simulink model "ieee80211n"  (Simulink 6.0)
settings: Solver=VariableStepDiscrete  StartTime=0.0  StopTime=inf  RelTol=1e-3
PreLoadFcn:
  | load IEEE80211n_init;
values from neighbouring files (symbols this model uses):
  params =     [IEEE80211n_init.mat]    (also in IEEE80211n_settings.m = p)
undefined symbols (not defined in the file or in its folder): magnitude
libraries: commblkintrlv2 x196, dspsigops x143, simulink x136, commdigbbndam2 x98, dspmtrx3 x96, dspsigattribs x69, dspstat3 x38, commutil2 x32, commsequence2 x26, commcnvcod2 x10, dspindex x9, dspmlti3 x8
(part 10 of 12)

== system ieee80211n/ModulatorBank/ModulatorSS1/Modulator 6 ==
  txdata : Inport  Port=1  LatchInput=off
  Enable : EnablePort
  Gain1 : Gain  SaturateOnIntegerOverflow=on
  General Block Interleaver : commblkintrlv2/General Block Interleaver  elements=interleaverElements
  Matrix Interleaver : commblkintrlv2/Matrix Interleaver  Nrows=interleaverRows  Ncols=interleaverCols
  Rectangular QAM Modulator Baseband : commdigbbndam2/Rectangular QAM Modulator Baseband  M=modOrder  InType=Bit  Enc=Gray  PowType=Average Power  MinDist=2  AvgPow=1  PeakPow=1  Ph=0  numSamp=1
  Zero Pad : dspsigops/Zero Pad  padSigAt=End  zpadAlong=Columns  padNumOutRowsSpecMethod=User-specified  numOutRows=Nb  padNumOutColsSpecMethod=User-specified  numOutCols=1  trunc_flag=None
      settings: AttributesFormatString=\n
  txsig : Outport
  wires:
  Rectangular QAM Modulator Baseband/1 -> Gain1/1
  Gain1/1 -> txsig/1
  txdata/1 -> Zero Pad/1
  Zero Pad/1 -> Matrix Interleaver/1
  Matrix Interleaver/1 -> General Block Interleaver/1
  General Block Interleaver/1 -> Rectangular QAM Modulator Baseband/1

== system ieee80211n/ModulatorBank/ModulatorSS1/Modulator 7 ==
  txdata : Inport  Port=1  LatchInput=off
  Enable : EnablePort
  Gain1 : Gain  SaturateOnIntegerOverflow=on
  General Block Interleaver : commblkintrlv2/General Block Interleaver  elements=interleaverElements
  Matrix Interleaver : commblkintrlv2/Matrix Interleaver  Nrows=interleaverRows  Ncols=interleaverCols
  Rectangular QAM Modulator Baseband : commdigbbndam2/Rectangular QAM Modulator Baseband  M=modOrder  InType=Bit  Enc=Gray  PowType=Average Power  MinDist=2  AvgPow=1  PeakPow=1  Ph=0  numSamp=1
  Zero Pad : dspsigops/Zero Pad  padSigAt=End  zpadAlong=Columns  padNumOutRowsSpecMethod=User-specified  numOutRows=Nb  padNumOutColsSpecMethod=User-specified  numOutCols=1  trunc_flag=None
      settings: AttributesFormatString=\n
  txsig : Outport
  wires:
  Rectangular QAM Modulator Baseband/1 -> Gain1/1
  Gain1/1 -> txsig/1
  txdata/1 -> Zero Pad/1
  Zero Pad/1 -> Matrix Interleaver/1
  Matrix Interleaver/1 -> General Block Interleaver/1
  General Block Interleaver/1 -> Rectangular QAM Modulator Baseband/1

== system ieee80211n/ModulatorBank/ModulatorSS1/Modulator 8 ==
  txdata : Inport  Port=1  LatchInput=off
  Enable : EnablePort
  Gain1 : Gain  SaturateOnIntegerOverflow=on
  General Block Interleaver : commblkintrlv2/General Block Interleaver  elements=interleaverElements
  Matrix Interleaver : commblkintrlv2/Matrix Interleaver  Nrows=interleaverRows  Ncols=interleaverCols
  Rectangular QAM Modulator Baseband : commdigbbndam2/Rectangular QAM Modulator Baseband  M=modOrder  InType=Bit  Enc=Gray  PowType=Average Power  MinDist=2  AvgPow=1  PeakPow=1  Ph=0  numSamp=1
  Zero Pad : dspsigops/Zero Pad  padSigAt=End  zpadAlong=Columns  padNumOutRowsSpecMethod=User-specified  numOutRows=Nb  padNumOutColsSpecMethod=User-specified  numOutCols=1  trunc_flag=None
      settings: AttributesFormatString=\n
  txsig : Outport
  wires:
  Rectangular QAM Modulator Baseband/1 -> Gain1/1
  Gain1/1 -> txsig/1
  txdata/1 -> Zero Pad/1
  Zero Pad/1 -> Matrix Interleaver/1
  Matrix Interleaver/1 -> General Block Interleaver/1
  General Block Interleaver/1 -> Rectangular QAM Modulator Baseband/1

== system ieee80211n/ModulatorBank/ModulatorSS2/Modulator 1 ==
  txdata : Inport  Port=1  LatchInput=off
  Enable : EnablePort
  Gain1 : Gain  SaturateOnIntegerOverflow=on
  General Block Interleaver : commblkintrlv2/General Block Interleaver  elements=interleaverElements
  General Block Interleaver1 : S-Function  AncestorBlock=commblkintrlv2/General Block Interleaver  FunctionName=scominterl  Parameters=elements,method  mask(General Block Interleaver){elements=freqRotInterleaverElements}
      mask help: Reorder the elements of the input vector. y = u(Elements). The length of Elements must match the input signal width.
      mask init:
      | method = 1;
      | commblkinterl(elements);
      mask Help: helpview(commbhelp)
      mask Display: disp('Frequency\nRotation\nInterleaver')
  Matrix Interleaver : commblkintrlv2/Matrix Interleaver  Nrows=interleaverRows  Ncols=interleaverCols
  Rectangular QAM Modulator Baseband : commdigbbndam2/Rectangular QAM Modulator Baseband  M=modOrder  InType=Bit  Enc=Gray  PowType=Average Power  MinDist=2  AvgPow=1  PeakPow=1  Ph=0  numSamp=1
  Zero Pad : dspsigops/Zero Pad  padSigAt=End  zpadAlong=Columns  padNumOutRowsSpecMethod=User-specified  numOutRows=Nb  padNumOutColsSpecMethod=User-specified  numOutCols=1  trunc_flag=None
      settings: AttributesFormatString=\n
  txsig : Outport
  wires:
  Rectangular QAM Modulator Baseband/1 -> Gain1/1
  Gain1/1 -> txsig/1
  txdata/1 -> Zero Pad/1
  Zero Pad/1 -> Matrix Interleaver/1
  Matrix Interleaver/1 -> General Block Interleaver/1
  General Block Interleaver/1 -> General Block Interleaver1/1
  General Block Interleaver1/1 -> Rectangular QAM Modulator Baseband/1

== system ieee80211n/ModulatorBank/ModulatorSS2/Modulator 2 ==
  txdata : Inport  Port=1  LatchInput=off
  Enable : EnablePort
  Gain1 : Gain  SaturateOnIntegerOverflow=on
  General Block Interleaver : commblkintrlv2/General Block Interleaver  elements=interleaverElements
  General Block Interleaver1 : S-Function  AncestorBlock=commblkintrlv2/General Block Interleaver  FunctionName=scominterl  Parameters=elements,method  mask(General Block Interleaver){elements=freqRotInterleaverElements}
      mask help: Reorder the elements of the input vector. y = u(Elements). The length of Elements must match the input signal width.
      mask init:
      | method = 1;
      | commblkinterl(elements);
      mask Help: helpview(commbhelp)
      mask Display: disp('Frequency\nRotation\nInterleaver')
  Matrix Interleaver : commblkintrlv2/Matrix Interleaver  Nrows=interleaverRows  Ncols=interleaverCols
  Rectangular QAM Modulator Baseband : commdigbbndam2/Rectangular QAM Modulator Baseband  M=modOrder  InType=Bit  Enc=Gray  PowType=Average Power  MinDist=2  AvgPow=1  PeakPow=1  Ph=0  numSamp=1
  Zero Pad : dspsigops/Zero Pad  padSigAt=End  zpadAlong=Columns  padNumOutRowsSpecMethod=User-specified  numOutRows=Nb  padNumOutColsSpecMethod=User-specified  numOutCols=1  trunc_flag=None
      settings: AttributesFormatString=\n
  txsig : Outport
  wires:
  Rectangular QAM Modulator Baseband/1 -> Gain1/1
  Gain1/1 -> txsig/1
  txdata/1 -> Zero Pad/1
  Zero Pad/1 -> Matrix Interleaver/1
  Matrix Interleaver/1 -> General Block Interleaver/1
  General Block Interleaver/1 -> General Block Interleaver1/1
  General Block Interleaver1/1 -> Rectangular QAM Modulator Baseband/1

== system ieee80211n/ModulatorBank/ModulatorSS2/Modulator 3 ==
  txdata : Inport  Port=1  LatchInput=off
  Enable : EnablePort
  Gain1 : Gain  SaturateOnIntegerOverflow=on
  General Block Interleaver : commblkintrlv2/General Block Interleaver  elements=interleaverElements
  General Block Interleaver1 : S-Function  AncestorBlock=commblkintrlv2/General Block Interleaver  FunctionName=scominterl  Parameters=elements,method  mask(General Block Interleaver){elements=freqRotInterleaverElements}
      mask help: Reorder the elements of the input vector. y = u(Elements). The length of Elements must match the input signal width.
      mask init:
      | method = 1;
      | commblkinterl(elements);
      mask Help: helpview(commbhelp)
      mask Display: disp('Frequency\nRotation\nInterleaver')
  Matrix Interleaver : commblkintrlv2/Matrix Interleaver  Nrows=interleaverRows  Ncols=interleaverCols
  Rectangular QAM Modulator Baseband : commdigbbndam2/Rectangular QAM Modulator Baseband  M=modOrder  InType=Bit  Enc=Gray  PowType=Average Power  MinDist=2  AvgPow=1  PeakPow=1  Ph=0  numSamp=1
  Zero Pad : dspsigops/Zero Pad  padSigAt=End  zpadAlong=Columns  padNumOutRowsSpecMethod=User-specified  numOutRows=Nb  padNumOutColsSpecMethod=User-specified  numOutCols=1  trunc_flag=None
      settings: AttributesFormatString=\n
  txsig : Outport
  wires:
  Rectangular QAM Modulator Baseband/1 -> Gain1/1
  Gain1/1 -> txsig/1
  txdata/1 -> Zero Pad/1
  Zero Pad/1 -> Matrix Interleaver/1
  Matrix Interleaver/1 -> General Block Interleaver/1
  General Block Interleaver/1 -> General Block Interleaver1/1
  General Block Interleaver1/1 -> Rectangular QAM Modulator Baseband/1

== system ieee80211n/ModulatorBank/ModulatorSS2/Modulator 4 ==
  txdata : Inport  Port=1  LatchInput=off
  Enable : EnablePort
  Gain1 : Gain  SaturateOnIntegerOverflow=on
  General Block Interleaver : commblkintrlv2/General Block Interleaver  elements=interleaverElements
  General Block Interleaver1 : S-Function  AncestorBlock=commblkintrlv2/General Block Interleaver  FunctionName=scominterl  Parameters=elements,method  mask(General Block Interleaver){elements=freqRotInterleaverElements}
      mask help: Reorder the elements of the input vector. y = u(Elements). The length of Elements must match the input signal width.
      mask init:
      | method = 1;
      | commblkinterl(elements);
      mask Help: helpview(commbhelp)
      mask Display: disp('Frequency\nRotation\nInterleaver')
  Matrix Interleaver : commblkintrlv2/Matrix Interleaver  Nrows=interleaverRows  Ncols=interleaverCols
  Rectangular QAM Modulator Baseband : commdigbbndam2/Rectangular QAM Modulator Baseband  M=modOrder  InType=Bit  Enc=Gray  PowType=Average Power  MinDist=2  AvgPow=1  PeakPow=1  Ph=0  numSamp=1
  Zero Pad : dspsigops/Zero Pad  padSigAt=End  zpadAlong=Columns  padNumOutRowsSpecMethod=User-specified  numOutRows=Nb  padNumOutColsSpecMethod=User-specified  numOutCols=1  trunc_flag=None
      settings: AttributesFormatString=\n
  txsig : Outport
  wires:
  Rectangular QAM Modulator Baseband/1 -> Gain1/1
  Gain1/1 -> txsig/1
  txdata/1 -> Zero Pad/1
  Zero Pad/1 -> Matrix Interleaver/1
  Matrix Interleaver/1 -> General Block Interleaver/1
  General Block Interleaver/1 -> General Block Interleaver1/1
  General Block Interleaver1/1 -> Rectangular QAM Modulator Baseband/1

== system ieee80211n/ModulatorBank/ModulatorSS2/Modulator 5 ==
  txdata : Inport  Port=1  LatchInput=off
  Enable : EnablePort
  Gain1 : Gain  SaturateOnIntegerOverflow=on
  General Block Interleaver : commblkintrlv2/General Block Interleaver  elements=interleaverElements
  General Block Interleaver1 : S-Function  AncestorBlock=commblkintrlv2/General Block Interleaver  FunctionName=scominterl  Parameters=elements,method  mask(General Block Interleaver){elements=freqRotInterleaverElements}
      mask help: Reorder the elements of the input vector. y = u(Elements). The length of Elements must match the input signal width.
      mask init:
      | method = 1;
      | commblkinterl(elements);
      mask Help: helpview(commbhelp)
      mask Display: disp('Frequency\nRotation\nInterleaver')
  Matrix Interleaver : commblkintrlv2/Matrix Interleaver  Nrows=interleaverRows  Ncols=interleaverCols
  Rectangular QAM Modulator Baseband : commdigbbndam2/Rectangular QAM Modulator Baseband  M=modOrder  InType=Bit  Enc=Gray  PowType=Average Power  MinDist=2  AvgPow=1  PeakPow=1  Ph=0  numSamp=1
  Zero Pad : dspsigops/Zero Pad  padSigAt=End  zpadAlong=Columns  padNumOutRowsSpecMethod=User-specified  numOutRows=Nb  padNumOutColsSpecMethod=User-specified  numOutCols=1  trunc_flag=None
      settings: AttributesFormatString=\n
  txsig : Outport
  wires:
  Rectangular QAM Modulator Baseband/1 -> Gain1/1
  Gain1/1 -> txsig/1
  txdata/1 -> Zero Pad/1
  Zero Pad/1 -> Matrix Interleaver/1
  Matrix Interleaver/1 -> General Block Interleaver/1
  General Block Interleaver/1 -> General Block Interleaver1/1
  General Block Interleaver1/1 -> Rectangular QAM Modulator Baseband/1

== system ieee80211n/ModulatorBank/ModulatorSS2/Modulator 6 ==
  txdata : Inport  Port=1  LatchInput=off
  Enable : EnablePort
  Gain1 : Gain  SaturateOnIntegerOverflow=on
  General Block Interleaver : commblkintrlv2/General Block Interleaver  elements=interleaverElements
  General Block Interleaver1 : S-Function  AncestorBlock=commblkintrlv2/General Block Interleaver  FunctionName=scominterl  Parameters=elements,method  mask(General Block Interleaver){elements=freqRotInterleaverElements}
      mask help: Reorder the elements of the input vector. y = u(Elements). The length of Elements must match the input signal width.
      mask init:
      | method = 1;
      | commblkinterl(elements);
      mask Help: helpview(commbhelp)
      mask Display: disp('Frequency\nRotation\nInterleaver')
  Matrix Interleaver : commblkintrlv2/Matrix Interleaver  Nrows=interleaverRows  Ncols=interleaverCols
  Rectangular QAM Modulator Baseband : commdigbbndam2/Rectangular QAM Modulator Baseband  M=modOrder  InType=Bit  Enc=Gray  PowType=Average Power  MinDist=2  AvgPow=1  PeakPow=1  Ph=0  numSamp=1
  Zero Pad : dspsigops/Zero Pad  padSigAt=End  zpadAlong=Columns  padNumOutRowsSpecMethod=User-specified  numOutRows=Nb  padNumOutColsSpecMethod=User-specified  numOutCols=1  trunc_flag=None
      settings: AttributesFormatString=\n
  txsig : Outport
  wires:
  Rectangular QAM Modulator Baseband/1 -> Gain1/1
  Gain1/1 -> txsig/1
  txdata/1 -> Zero Pad/1
  Zero Pad/1 -> Matrix Interleaver/1
  Matrix Interleaver/1 -> General Block Interleaver/1
  General Block Interleaver/1 -> General Block Interleaver1/1
  General Block Interleaver1/1 -> Rectangular QAM Modulator Baseband/1

== system ieee80211n/ModulatorBank/ModulatorSS2/Modulator 7 ==
  txdata : Inport  Port=1  LatchInput=off
  Enable : EnablePort
  Gain1 : Gain  SaturateOnIntegerOverflow=on
  General Block Interleaver : commblkintrlv2/General Block Interleaver  elements=interleaverElements
  General Block Interleaver1 : S-Function  AncestorBlock=commblkintrlv2/General Block Interleaver  FunctionName=scominterl  Parameters=elements,method  mask(General Block Interleaver){elements=freqRotInterleaverElements}
      mask help: Reorder the elements of the input vector. y = u(Elements). The length of Elements must match the input signal width.
      mask init:
      | method = 1;
      | commblkinterl(elements);
      mask Help: helpview(commbhelp)
      mask Display: disp('Frequency\nRotation\nInterleaver')
  Matrix Interleaver : commblkintrlv2/Matrix Interleaver  Nrows=interleaverRows  Ncols=interleaverCols
  Rectangular QAM Modulator Baseband : commdigbbndam2/Rectangular QAM Modulator Baseband  M=modOrder  InType=Bit  Enc=Gray  PowType=Average Power  MinDist=2  AvgPow=1  PeakPow=1  Ph=0  numSamp=1
  Zero Pad : dspsigops/Zero Pad  padSigAt=End  zpadAlong=Columns  padNumOutRowsSpecMethod=User-specified  numOutRows=Nb  padNumOutColsSpecMethod=User-specified  numOutCols=1  trunc_flag=None
      settings: AttributesFormatString=\n
  txsig : Outport
  wires:
  Rectangular QAM Modulator Baseband/1 -> Gain1/1
  Gain1/1 -> txsig/1
  txdata/1 -> Zero Pad/1
  Zero Pad/1 -> Matrix Interleaver/1
  Matrix Interleaver/1 -> General Block Interleaver/1
  General Block Interleaver/1 -> General Block Interleaver1/1
  General Block Interleaver1/1 -> Rectangular QAM Modulator Baseband/1

== system ieee80211n/ModulatorBank/ModulatorSS2/Modulator 8 ==
  txdata : Inport  Port=1  LatchInput=off
  Enable : EnablePort
  Gain1 : Gain  SaturateOnIntegerOverflow=on
  General Block Interleaver : commblkintrlv2/General Block Interleaver  elements=interleaverElements
  General Block Interleaver1 : S-Function  AncestorBlock=commblkintrlv2/General Block Interleaver  FunctionName=scominterl  Parameters=elements,method  mask(General Block Interleaver){elements=freqRotInterleaverElements}
      mask help: Reorder the elements of the input vector. y = u(Elements). The length of Elements must match the input signal width.
      mask init:
      | method = 1;
      | commblkinterl(elements);
      mask Help: helpview(commbhelp)
      mask Display: disp('Frequency\nRotation\nInterleaver')
  Matrix Interleaver : commblkintrlv2/Matrix Interleaver  Nrows=interleaverRows  Ncols=interleaverCols
  Rectangular QAM Modulator Baseband : commdigbbndam2/Rectangular QAM Modulator Baseband  M=modOrder  InType=Bit  Enc=Gray  PowType=Average Power  MinDist=2  AvgPow=1  PeakPow=1  Ph=0  numSamp=1
  Zero Pad : dspsigops/Zero Pad  padSigAt=End  zpadAlong=Columns  padNumOutRowsSpecMethod=User-specified  numOutRows=Nb  padNumOutColsSpecMethod=User-specified  numOutCols=1  trunc_flag=None
      settings: AttributesFormatString=\n
  txsig : Outport
  wires:
  Rectangular QAM Modulator Baseband/1 -> Gain1/1
  Gain1/1 -> txsig/1
  txdata/1 -> Zero Pad/1
  Zero Pad/1 -> Matrix Interleaver/1
  Matrix Interleaver/1 -> General Block Interleaver/1
  General Block Interleaver/1 -> General Block Interleaver1/1
  General Block Interleaver1/1 -> Rectangular QAM Modulator Baseband/1

== system ieee80211n/ModulatorBank/ModulatorSS3/Modulator 1 ==
  txdata : Inport  Port=1  LatchInput=off
  Enable : EnablePort
  Gain1 : Gain  SaturateOnIntegerOverflow=on
  General Block Interleaver : commblkintrlv2/General Block Interleaver  elements=interleaverElements
  General Block Interleaver1 : S-Function  AncestorBlock=commblkintrlv2/General Block Interleaver  FunctionName=scominterl  Parameters=elements,method  mask(General Block Interleaver){elements=freqRotInterleaverElements}
      mask help: Reorder the elements of the input vector. y = u(Elements). The length of Elements must match the input signal width.
      mask init:
      | method = 1;
      | commblkinterl(elements);
      mask Help: helpview(commbhelp)
      mask Display: disp('Frequency\nRotation\nInterleaver')
  Matrix Interleaver : commblkintrlv2/Matrix Interleaver  Nrows=interleaverRows  Ncols=interleaverCols
  Rectangular QAM Modulator Baseband : commdigbbndam2/Rectangular QAM Modulator Baseband  M=modOrder  InType=Bit  Enc=Gray  PowType=Average Power  MinDist=2  AvgPow=1  PeakPow=1  Ph=0  numSamp=1
  Zero Pad : dspsigops/Zero Pad  padSigAt=End  zpadAlong=Columns  padNumOutRowsSpecMethod=User-specified  numOutRows=Nb  padNumOutColsSpecMethod=User-specified  numOutCols=1  trunc_flag=None
      settings: AttributesFormatString=\n
  txsig : Outport
  wires:
  Rectangular QAM Modulator Baseband/1 -> Gain1/1
  Gain1/1 -> txsig/1
  txdata/1 -> Zero Pad/1
  Zero Pad/1 -> Matrix Interleaver/1
  Matrix Interleaver/1 -> General Block Interleaver/1
  General Block Interleaver/1 -> General Block Interleaver1/1
  General Block Interleaver1/1 -> Rectangular QAM Modulator Baseband/1

== system ieee80211n/ModulatorBank/ModulatorSS3/Modulator 2 ==
  txdata : Inport  Port=1  LatchInput=off
  Enable : EnablePort
  Gain1 : Gain  SaturateOnIntegerOverflow=on
  General Block Interleaver : commblkintrlv2/General Block Interleaver  elements=interleaverElements
  General Block Interleaver1 : S-Function  AncestorBlock=commblkintrlv2/General Block Interleaver  FunctionName=scominterl  Parameters=elements,method  mask(General Block Interleaver){elements=freqRotInterleaverElements}
      mask help: Reorder the elements of the input vector. y = u(Elements). The length of Elements must match the input signal width.
      mask init:
      | method = 1;
      | commblkinterl(elements);
      mask Help: helpview(commbhelp)
      mask Display: disp('Frequency\nRotation\nInterleaver')
  Matrix Interleaver : commblkintrlv2/Matrix Interleaver  Nrows=interleaverRows  Ncols=interleaverCols
  Rectangular QAM Modulator Baseband : commdigbbndam2/Rectangular QAM Modulator Baseband  M=modOrder  InType=Bit  Enc=Gray  PowType=Average Power  MinDist=2  AvgPow=1  PeakPow=1  Ph=0  numSamp=1
  Zero Pad : dspsigops/Zero Pad  padSigAt=End  zpadAlong=Columns  padNumOutRowsSpecMethod=User-specified  numOutRows=Nb  padNumOutColsSpecMethod=User-specified  numOutCols=1  trunc_flag=None
      settings: AttributesFormatString=\n
  txsig : Outport
  wires:
  Rectangular QAM Modulator Baseband/1 -> Gain1/1
  Gain1/1 -> txsig/1
  txdata/1 -> Zero Pad/1
  Zero Pad/1 -> Matrix Interleaver/1
  Matrix Interleaver/1 -> General Block Interleaver/1
  General Block Interleaver/1 -> General Block Interleaver1/1
  General Block Interleaver1/1 -> Rectangular QAM Modulator Baseband/1

== system ieee80211n/ModulatorBank/ModulatorSS3/Modulator 3 ==
  txdata : Inport  Port=1  LatchInput=off
  Enable : EnablePort
  Gain1 : Gain  SaturateOnIntegerOverflow=on
  General Block Interleaver : commblkintrlv2/General Block Interleaver  elements=interleaverElements
  General Block Interleaver1 : S-Function  AncestorBlock=commblkintrlv2/General Block Interleaver  FunctionName=scominterl  Parameters=elements,method  mask(General Block Interleaver){elements=freqRotInterleaverElements}
      mask help: Reorder the elements of the input vector. y = u(Elements). The length of Elements must match the input signal width.
      mask init:
      | method = 1;
      | commblkinterl(elements);
      mask Help: helpview(commbhelp)
      mask Display: disp('Frequency\nRotation\nInterleaver')
  Matrix Interleaver : commblkintrlv2/Matrix Interleaver  Nrows=interleaverRows  Ncols=interleaverCols
  Rectangular QAM Modulator Baseband : commdigbbndam2/Rectangular QAM Modulator Baseband  M=modOrder  InType=Bit  Enc=Gray  PowType=Average Power  MinDist=2  AvgPow=1  PeakPow=1  Ph=0  numSamp=1
  Zero Pad : dspsigops/Zero Pad  padSigAt=End  zpadAlong=Columns  padNumOutRowsSpecMethod=User-specified  numOutRows=Nb  padNumOutColsSpecMethod=User-specified  numOutCols=1  trunc_flag=None
      settings: AttributesFormatString=\n
  txsig : Outport
  wires:
  Rectangular QAM Modulator Baseband/1 -> Gain1/1
  Gain1/1 -> txsig/1
  txdata/1 -> Zero Pad/1
  Zero Pad/1 -> Matrix Interleaver/1
  Matrix Interleaver/1 -> General Block Interleaver/1
  General Block Interleaver/1 -> General Block Interleaver1/1
  General Block Interleaver1/1 -> Rectangular QAM Modulator Baseband/1

== system ieee80211n/ModulatorBank/ModulatorSS3/Modulator 4 ==
  txdata : Inport  Port=1  LatchInput=off
  Enable : EnablePort
  Gain1 : Gain  SaturateOnIntegerOverflow=on
  General Block Interleaver : commblkintrlv2/General Block Interleaver  elements=interleaverElements
  General Block Interleaver1 : S-Function  AncestorBlock=commblkintrlv2/General Block Interleaver  FunctionName=scominterl  Parameters=elements,method  mask(General Block Interleaver){elements=freqRotInterleaverElements}
      mask help: Reorder the elements of the input vector. y = u(Elements). The length of Elements must match the input signal width.
      mask init:
      | method = 1;
      | commblkinterl(elements);
      mask Help: helpview(commbhelp)
      mask Display: disp('Frequency\nRotation\nInterleaver')
  Matrix Interleaver : commblkintrlv2/Matrix Interleaver  Nrows=interleaverRows  Ncols=interleaverCols
  Rectangular QAM Modulator Baseband : commdigbbndam2/Rectangular QAM Modulator Baseband  M=modOrder  InType=Bit  Enc=Gray  PowType=Average Power  MinDist=2  AvgPow=1  PeakPow=1  Ph=0  numSamp=1
  Zero Pad : dspsigops/Zero Pad  padSigAt=End  zpadAlong=Columns  padNumOutRowsSpecMethod=User-specified  numOutRows=Nb  padNumOutColsSpecMethod=User-specified  numOutCols=1  trunc_flag=None
      settings: AttributesFormatString=\n
  txsig : Outport
  wires:
  Rectangular QAM Modulator Baseband/1 -> Gain1/1
  Gain1/1 -> txsig/1
  txdata/1 -> Zero Pad/1
  Zero Pad/1 -> Matrix Interleaver/1
  Matrix Interleaver/1 -> General Block Interleaver/1
  General Block Interleaver/1 -> General Block Interleaver1/1
  General Block Interleaver1/1 -> Rectangular QAM Modulator Baseband/1

== system ieee80211n/ModulatorBank/ModulatorSS3/Modulator 5 ==
  txdata : Inport  Port=1  LatchInput=off
  Enable : EnablePort
  Gain1 : Gain  SaturateOnIntegerOverflow=on
  General Block Interleaver : commblkintrlv2/General Block Interleaver  elements=interleaverElements
  General Block Interleaver1 : S-Function  AncestorBlock=commblkintrlv2/General Block Interleaver  FunctionName=scominterl  Parameters=elements,method  mask(General Block Interleaver){elements=freqRotInterleaverElements}
      mask help: Reorder the elements of the input vector. y = u(Elements). The length of Elements must match the input signal width.
      mask init:
      | method = 1;
      | commblkinterl(elements);
      mask Help: helpview(commbhelp)
      mask Display: disp('Frequency\nRotation\nInterleaver')
  Matrix Interleaver : commblkintrlv2/Matrix Interleaver  Nrows=interleaverRows  Ncols=interleaverCols
  Rectangular QAM Modulator Baseband : commdigbbndam2/Rectangular QAM Modulator Baseband  M=modOrder  InType=Bit  Enc=Gray  PowType=Average Power  MinDist=2  AvgPow=1  PeakPow=1  Ph=0  numSamp=1
  Zero Pad : dspsigops/Zero Pad  padSigAt=End  zpadAlong=Columns  padNumOutRowsSpecMethod=User-specified  numOutRows=Nb  padNumOutColsSpecMethod=User-specified  numOutCols=1  trunc_flag=None
      settings: AttributesFormatString=\n
  txsig : Outport
  wires:
  Rectangular QAM Modulator Baseband/1 -> Gain1/1
  Gain1/1 -> txsig/1
  txdata/1 -> Zero Pad/1
  Zero Pad/1 -> Matrix Interleaver/1
  Matrix Interleaver/1 -> General Block Interleaver/1
  General Block Interleaver/1 -> General Block Interleaver1/1
  General Block Interleaver1/1 -> Rectangular QAM Modulator Baseband/1

== system ieee80211n/ModulatorBank/ModulatorSS3/Modulator 6 ==
  txdata : Inport  Port=1  LatchInput=off
  Enable : EnablePort
  Gain1 : Gain  SaturateOnIntegerOverflow=on
  General Block Interleaver : commblkintrlv2/General Block Interleaver  elements=interleaverElements
  General Block Interleaver1 : S-Function  AncestorBlock=commblkintrlv2/General Block Interleaver  FunctionName=scominterl  Parameters=elements,method  mask(General Block Interleaver){elements=freqRotInterleaverElements}
      mask help: Reorder the elements of the input vector. y = u(Elements). The length of Elements must match the input signal width.
      mask init:
      | method = 1;
      | commblkinterl(elements);
      mask Help: helpview(commbhelp)
      mask Display: disp('Frequency\nRotation\nInterleaver')
  Matrix Interleaver : commblkintrlv2/Matrix Interleaver  Nrows=interleaverRows  Ncols=interleaverCols
  Rectangular QAM Modulator Baseband : commdigbbndam2/Rectangular QAM Modulator Baseband  M=modOrder  InType=Bit  Enc=Gray  PowType=Average Power  MinDist=2  AvgPow=1  PeakPow=1  Ph=0  numSamp=1
  Zero Pad : dspsigops/Zero Pad  padSigAt=End  zpadAlong=Columns  padNumOutRowsSpecMethod=User-specified  numOutRows=Nb  padNumOutColsSpecMethod=User-specified  numOutCols=1  trunc_flag=None
      settings: AttributesFormatString=\n
  txsig : Outport
  wires:
  Rectangular QAM Modulator Baseband/1 -> Gain1/1
  Gain1/1 -> txsig/1
  txdata/1 -> Zero Pad/1
  Zero Pad/1 -> Matrix Interleaver/1
  Matrix Interleaver/1 -> General Block Interleaver/1
  General Block Interleaver/1 -> General Block Interleaver1/1
  General Block Interleaver1/1 -> Rectangular QAM Modulator Baseband/1

== system ieee80211n/ModulatorBank/ModulatorSS3/Modulator 7 ==
  txdata : Inport  Port=1  LatchInput=off
  Enable : EnablePort
  Gain1 : Gain  SaturateOnIntegerOverflow=on
  General Block Interleaver : commblkintrlv2/General Block Interleaver  elements=interleaverElements
  General Block Interleaver1 : S-Function  AncestorBlock=commblkintrlv2/General Block Interleaver  FunctionName=scominterl  Parameters=elements,method  mask(General Block Interleaver){elements=freqRotInterleaverElements}
      mask help: Reorder the elements of the input vector. y = u(Elements). The length of Elements must match the input signal width.
      mask init:
      | method = 1;
      | commblkinterl(elements);
      mask Help: helpview(commbhelp)
      mask Display: disp('Frequency\nRotation\nInterleaver')
  Matrix Interleaver : commblkintrlv2/Matrix Interleaver  Nrows=interleaverRows  Ncols=interleaverCols
  Rectangular QAM Modulator Baseband : commdigbbndam2/Rectangular QAM Modulator Baseband  M=modOrder  InType=Bit  Enc=Gray  PowType=Average Power  MinDist=2  AvgPow=1  PeakPow=1  Ph=0  numSamp=1
  Zero Pad : dspsigops/Zero Pad  padSigAt=End  zpadAlong=Columns  padNumOutRowsSpecMethod=User-specified  numOutRows=Nb  padNumOutColsSpecMethod=User-specified  numOutCols=1  trunc_flag=None
      settings: AttributesFormatString=\n
  txsig : Outport
  wires:
  Rectangular QAM Modulator Baseband/1 -> Gain1/1
  Gain1/1 -> txsig/1
  txdata/1 -> Zero Pad/1
  Zero Pad/1 -> Matrix Interleaver/1
  Matrix Interleaver/1 -> General Block Interleaver/1
  General Block Interleaver/1 -> General Block Interleaver1/1
  General Block Interleaver1/1 -> Rectangular QAM Modulator Baseband/1

== system ieee80211n/ModulatorBank/ModulatorSS3/Modulator 8 ==
  txdata : Inport  Port=1  LatchInput=off
  Enable : EnablePort
  Gain1 : Gain  SaturateOnIntegerOverflow=on
  General Block Interleaver : commblkintrlv2/General Block Interleaver  elements=interleaverElements
  General Block Interleaver1 : S-Function  AncestorBlock=commblkintrlv2/General Block Interleaver  FunctionName=scominterl  Parameters=elements,method  mask(General Block Interleaver){elements=freqRotInterleaverElements}
      mask help: Reorder the elements of the input vector. y = u(Elements). The length of Elements must match the input signal width.
      mask init:
      | method = 1;
      | commblkinterl(elements);
      mask Help: helpview(commbhelp)
      mask Display: disp('Frequency\nRotation\nInterleaver')
  Matrix Interleaver : commblkintrlv2/Matrix Interleaver  Nrows=interleaverRows  Ncols=interleaverCols
  Rectangular QAM Modulator Baseband : commdigbbndam2/Rectangular QAM Modulator Baseband  M=modOrder  InType=Bit  Enc=Gray  PowType=Average Power  MinDist=2  AvgPow=1  PeakPow=1  Ph=0  numSamp=1
  Zero Pad : dspsigops/Zero Pad  padSigAt=End  zpadAlong=Columns  padNumOutRowsSpecMethod=User-specified  numOutRows=Nb  padNumOutColsSpecMethod=User-specified  numOutCols=1  trunc_flag=None
      settings: AttributesFormatString=\n
  txsig : Outport
  wires:
  Rectangular QAM Modulator Baseband/1 -> Gain1/1
  Gain1/1 -> txsig/1
  txdata/1 -> Zero Pad/1
  Zero Pad/1 -> Matrix Interleaver/1
  Matrix Interleaver/1 -> General Block Interleaver/1
  General Block Interleaver/1 -> General Block Interleaver1/1
  General Block Interleaver1/1 -> Rectangular QAM Modulator Baseband/1

== system ieee80211n/ModulatorBank/ModulatorSS4/Modulator 1 ==
  txdata : Inport  Port=1  LatchInput=off
  Enable : EnablePort
  Gain1 : Gain  SaturateOnIntegerOverflow=on
  General Block Interleaver : commblkintrlv2/General Block Interleaver  elements=interleaverElements
  General Block Interleaver1 : S-Function  AncestorBlock=commblkintrlv2/General Block Interleaver  FunctionName=scominterl  Parameters=elements,method  mask(General Block Interleaver){elements=freqRotInterleaverElements}
      mask help: Reorder the elements of the input vector. y = u(Elements). The length of Elements must match the input signal width.
      mask init:
      | method = 1;
      | commblkinterl(elements);
      mask Help: helpview(commbhelp)
      mask Display: disp('Frequency\nRotation\nInterleaver')
  Matrix Interleaver : commblkintrlv2/Matrix Interleaver  Nrows=interleaverRows  Ncols=interleaverCols
  Rectangular QAM Modulator Baseband : commdigbbndam2/Rectangular QAM Modulator Baseband  M=modOrder  InType=Bit  Enc=Gray  PowType=Average Power  MinDist=2  AvgPow=1  PeakPow=1  Ph=0  numSamp=1
  Zero Pad : dspsigops/Zero Pad  padSigAt=End  zpadAlong=Columns  padNumOutRowsSpecMethod=User-specified  numOutRows=Nb  padNumOutColsSpecMethod=User-specified  numOutCols=1  trunc_flag=None
      settings: AttributesFormatString=\n
  txsig : Outport
  wires:
  Rectangular QAM Modulator Baseband/1 -> Gain1/1
  Gain1/1 -> txsig/1
  txdata/1 -> Zero Pad/1
  Zero Pad/1 -> Matrix Interleaver/1
  Matrix Interleaver/1 -> General Block Interleaver/1
  General Block Interleaver/1 -> General Block Interleaver1/1
  General Block Interleaver1/1 -> Rectangular QAM Modulator Baseband/1

== system ieee80211n/ModulatorBank/ModulatorSS4/Modulator 2 ==
  txdata : Inport  Port=1  LatchInput=off
  Enable : EnablePort
  Gain1 : Gain  SaturateOnIntegerOverflow=on
  General Block Interleaver : commblkintrlv2/General Block Interleaver  elements=interleaverElements
  General Block Interleaver1 : S-Function  AncestorBlock=commblkintrlv2/General Block Interleaver  FunctionName=scominterl  Parameters=elements,method  mask(General Block Interleaver){elements=freqRotInterleaverElements}
      mask help: Reorder the elements of the input vector. y = u(Elements). The length of Elements must match the input signal width.
      mask init:
      | method = 1;
      | commblkinterl(elements);
      mask Help: helpview(commbhelp)
      mask Display: disp('Frequency\nRotation\nInterleaver')
  Matrix Interleaver : commblkintrlv2/Matrix Interleaver  Nrows=interleaverRows  Ncols=interleaverCols
  Rectangular QAM Modulator Baseband : commdigbbndam2/Rectangular QAM Modulator Baseband  M=modOrder  InType=Bit  Enc=Gray  PowType=Average Power  MinDist=2  AvgPow=1  PeakPow=1  Ph=0  numSamp=1
  Zero Pad : dspsigops/Zero Pad  padSigAt=End  zpadAlong=Columns  padNumOutRowsSpecMethod=User-specified  numOutRows=Nb  padNumOutColsSpecMethod=User-specified  numOutCols=1  trunc_flag=None
      settings: AttributesFormatString=\n
  txsig : Outport
  wires:
  Rectangular QAM Modulator Baseband/1 -> Gain1/1
  Gain1/1 -> txsig/1
  txdata/1 -> Zero Pad/1
  Zero Pad/1 -> Matrix Interleaver/1
  Matrix Interleaver/1 -> General Block Interleaver/1
  General Block Interleaver/1 -> General Block Interleaver1/1
  General Block Interleaver1/1 -> Rectangular QAM Modulator Baseband/1

== system ieee80211n/ModulatorBank/ModulatorSS4/Modulator 3 ==
  txdata : Inport  Port=1  LatchInput=off
  Enable : EnablePort
  Gain1 : Gain  SaturateOnIntegerOverflow=on
  General Block Interleaver : commblkintrlv2/General Block Interleaver  elements=interleaverElements
  General Block Interleaver1 : S-Function  AncestorBlock=commblkintrlv2/General Block Interleaver  FunctionName=scominterl  Parameters=elements,method  mask(General Block Interleaver){elements=freqRotInterleaverElements}
      mask help: Reorder the elements of the input vector. y = u(Elements). The length of Elements must match the input signal width.
      mask init:
      | method = 1;
      | commblkinterl(elements);
      mask Help: helpview(commbhelp)
      mask Display: disp('Frequency\nRotation\nInterleaver')
  Matrix Interleaver : commblkintrlv2/Matrix Interleaver  Nrows=interleaverRows  Ncols=interleaverCols
  Rectangular QAM Modulator Baseband : commdigbbndam2/Rectangular QAM Modulator Baseband  M=modOrder  InType=Bit  Enc=Gray  PowType=Average Power  MinDist=2  AvgPow=1  PeakPow=1  Ph=0  numSamp=1
  Zero Pad : dspsigops/Zero Pad  padSigAt=End  zpadAlong=Columns  padNumOutRowsSpecMethod=User-specified  numOutRows=Nb  padNumOutColsSpecMethod=User-specified  numOutCols=1  trunc_flag=None
      settings: AttributesFormatString=\n
  txsig : Outport
  wires:
  Rectangular QAM Modulator Baseband/1 -> Gain1/1
  Gain1/1 -> txsig/1
  txdata/1 -> Zero Pad/1
  Zero Pad/1 -> Matrix Interleaver/1
  Matrix Interleaver/1 -> General Block Interleaver/1
  General Block Interleaver/1 -> General Block Interleaver1/1
  General Block Interleaver1/1 -> Rectangular QAM Modulator Baseband/1

== system ieee80211n/ModulatorBank/ModulatorSS4/Modulator 4 ==
  txdata : Inport  Port=1  LatchInput=off
  Enable : EnablePort
  Gain1 : Gain  SaturateOnIntegerOverflow=on
  General Block Interleaver : commblkintrlv2/General Block Interleaver  elements=interleaverElements
  General Block Interleaver1 : S-Function  AncestorBlock=commblkintrlv2/General Block Interleaver  FunctionName=scominterl  Parameters=elements,method  mask(General Block Interleaver){elements=freqRotInterleaverElements}
      mask help: Reorder the elements of the input vector. y = u(Elements). The length of Elements must match the input signal width.
      mask init:
      | method = 1;
      | commblkinterl(elements);
      mask Help: helpview(commbhelp)
      mask Display: disp('Frequency\nRotation\nInterleaver')
  Matrix Interleaver : commblkintrlv2/Matrix Interleaver  Nrows=interleaverRows  Ncols=interleaverCols
  Rectangular QAM Modulator Baseband : commdigbbndam2/Rectangular QAM Modulator Baseband  M=modOrder  InType=Bit  Enc=Gray  PowType=Average Power  MinDist=2  AvgPow=1  PeakPow=1  Ph=0  numSamp=1
  Zero Pad : dspsigops/Zero Pad  padSigAt=End  zpadAlong=Columns  padNumOutRowsSpecMethod=User-specified  numOutRows=Nb  padNumOutColsSpecMethod=User-specified  numOutCols=1  trunc_flag=None
      settings: AttributesFormatString=\n
  txsig : Outport
  wires:
  Rectangular QAM Modulator Baseband/1 -> Gain1/1
  Gain1/1 -> txsig/1
  txdata/1 -> Zero Pad/1
  Zero Pad/1 -> Matrix Interleaver/1
  Matrix Interleaver/1 -> General Block Interleaver/1
  General Block Interleaver/1 -> General Block Interleaver1/1
  General Block Interleaver1/1 -> Rectangular QAM Modulator Baseband/1

== system ieee80211n/ModulatorBank/ModulatorSS4/Modulator 5 ==
  txdata : Inport  Port=1  LatchInput=off
  Enable : EnablePort
  Gain1 : Gain  SaturateOnIntegerOverflow=on
  General Block Interleaver : commblkintrlv2/General Block Interleaver  elements=interleaverElements
  General Block Interleaver1 : S-Function  AncestorBlock=commblkintrlv2/General Block Interleaver  FunctionName=scominterl  Parameters=elements,method  mask(General Block Interleaver){elements=freqRotInterleaverElements}
      mask help: Reorder the elements of the input vector. y = u(Elements). The length of Elements must match the input signal width.
      mask init:
      | method = 1;
      | commblkinterl(elements);
      mask Help: helpview(commbhelp)
      mask Display: disp('Frequency\nRotation\nInterleaver')
  Matrix Interleaver : commblkintrlv2/Matrix Interleaver  Nrows=interleaverRows  Ncols=interleaverCols
  Rectangular QAM Modulator Baseband : commdigbbndam2/Rectangular QAM Modulator Baseband  M=modOrder  InType=Bit  Enc=Gray  PowType=Average Power  MinDist=2  AvgPow=1  PeakPow=1  Ph=0  numSamp=1
  Zero Pad : dspsigops/Zero Pad  padSigAt=End  zpadAlong=Columns  padNumOutRowsSpecMethod=User-specified  numOutRows=Nb  padNumOutColsSpecMethod=User-specified  numOutCols=1  trunc_flag=None
      settings: AttributesFormatString=\n
  txsig : Outport
  wires:
  Rectangular QAM Modulator Baseband/1 -> Gain1/1
  Gain1/1 -> txsig/1
  txdata/1 -> Zero Pad/1
  Zero Pad/1 -> Matrix Interleaver/1
  Matrix Interleaver/1 -> General Block Interleaver/1
  General Block Interleaver/1 -> General Block Interleaver1/1
  General Block Interleaver1/1 -> Rectangular QAM Modulator Baseband/1

== system ieee80211n/ModulatorBank/ModulatorSS4/Modulator 6 ==
  txdata : Inport  Port=1  LatchInput=off
  Enable : EnablePort
  Gain1 : Gain  SaturateOnIntegerOverflow=on
  General Block Interleaver : commblkintrlv2/General Block Interleaver  elements=interleaverElements
  General Block Interleaver1 : S-Function  AncestorBlock=commblkintrlv2/General Block Interleaver  FunctionName=scominterl  Parameters=elements,method  mask(General Block Interleaver){elements=freqRotInterleaverElements}
      mask help: Reorder the elements of the input vector. y = u(Elements). The length of Elements must match the input signal width.
      mask init:
      | method = 1;
      | commblkinterl(elements);
      mask Help: helpview(commbhelp)
      mask Display: disp('Frequency\nRotation\nInterleaver')
  Matrix Interleaver : commblkintrlv2/Matrix Interleaver  Nrows=interleaverRows  Ncols=interleaverCols
  Rectangular QAM Modulator Baseband : commdigbbndam2/Rectangular QAM Modulator Baseband  M=modOrder  InType=Bit  Enc=Gray  PowType=Average Power  MinDist=2  AvgPow=1  PeakPow=1  Ph=0  numSamp=1
  Zero Pad : dspsigops/Zero Pad  padSigAt=End  zpadAlong=Columns  padNumOutRowsSpecMethod=User-specified  numOutRows=Nb  padNumOutColsSpecMethod=User-specified  numOutCols=1  trunc_flag=None
      settings: AttributesFormatString=\n
  txsig : Outport
  wires:
  Rectangular QAM Modulator Baseband/1 -> Gain1/1
  Gain1/1 -> txsig/1
  txdata/1 -> Zero Pad/1
  Zero Pad/1 -> Matrix Interleaver/1
  Matrix Interleaver/1 -> General Block Interleaver/1
  General Block Interleaver/1 -> General Block Interleaver1/1
  General Block Interleaver1/1 -> Rectangular QAM Modulator Baseband/1

== system ieee80211n/ModulatorBank/ModulatorSS4/Modulator 7 ==
  txdata : Inport  Port=1  LatchInput=off
  Enable : EnablePort
  Gain1 : Gain  SaturateOnIntegerOverflow=on
  General Block Interleaver : commblkintrlv2/General Block Interleaver  elements=interleaverElements
  General Block Interleaver1 : S-Function  AncestorBlock=commblkintrlv2/General Block Interleaver  FunctionName=scominterl  Parameters=elements,method  mask(General Block Interleaver){elements=freqRotInterleaverElements}
      mask help: Reorder the elements of the input vector. y = u(Elements). The length of Elements must match the input signal width.
      mask init:
      | method = 1;
      | commblkinterl(elements);
      mask Help: helpview(commbhelp)
      mask Display: disp('Frequency\nRotation\nInterleaver')
  Matrix Interleaver : commblkintrlv2/Matrix Interleaver  Nrows=interleaverRows  Ncols=interleaverCols
  Rectangular QAM Modulator Baseband : commdigbbndam2/Rectangular QAM Modulator Baseband  M=modOrder  InType=Bit  Enc=Gray  PowType=Average Power  MinDist=2  AvgPow=1  PeakPow=1  Ph=0  numSamp=1
  Zero Pad : dspsigops/Zero Pad  padSigAt=End  zpadAlong=Columns  padNumOutRowsSpecMethod=User-specified  numOutRows=Nb  padNumOutColsSpecMethod=User-specified  numOutCols=1  trunc_flag=None
      settings: AttributesFormatString=\n
  txsig : Outport
  wires:
  Rectangular QAM Modulator Baseband/1 -> Gain1/1
  Gain1/1 -> txsig/1
  txdata/1 -> Zero Pad/1
  Zero Pad/1 -> Matrix Interleaver/1
  Matrix Interleaver/1 -> General Block Interleaver/1
  General Block Interleaver/1 -> General Block Interleaver1/1
  General Block Interleaver1/1 -> Rectangular QAM Modulator Baseband/1

== system ieee80211n/ModulatorBank/ModulatorSS4/Modulator 8 ==
  txdata : Inport  Port=1  LatchInput=off
  Enable : EnablePort
  Gain1 : Gain  SaturateOnIntegerOverflow=on
  General Block Interleaver : commblkintrlv2/General Block Interleaver  elements=interleaverElements
  General Block Interleaver1 : S-Function  AncestorBlock=commblkintrlv2/General Block Interleaver  FunctionName=scominterl  Parameters=elements,method  mask(General Block Interleaver){elements=freqRotInterleaverElements}
      mask help: Reorder the elements of the input vector. y = u(Elements). The length of Elements must match the input signal width.
      mask init:
      | method = 1;
      | commblkinterl(elements);
      mask Help: helpview(commbhelp)
      mask Display: disp('Frequency\nRotation\nInterleaver')
  Matrix Interleaver : commblkintrlv2/Matrix Interleaver  Nrows=interleaverRows  Ncols=interleaverCols
  Rectangular QAM Modulator Baseband : commdigbbndam2/Rectangular QAM Modulator Baseband  M=modOrder  InType=Bit  Enc=Gray  PowType=Average Power  MinDist=2  AvgPow=1  PeakPow=1  Ph=0  numSamp=1
  Zero Pad : dspsigops/Zero Pad  padSigAt=End  zpadAlong=Columns  padNumOutRowsSpecMethod=User-specified  numOutRows=Nb  padNumOutColsSpecMethod=User-specified  numOutCols=1  trunc_flag=None
      settings: AttributesFormatString=\n
  txsig : Outport
  wires:
  Rectangular QAM Modulator Baseband/1 -> Gain1/1
  Gain1/1 -> txsig/1
  txdata/1 -> Zero Pad/1
  Zero Pad/1 -> Matrix Interleaver/1
  Matrix Interleaver/1 -> General Block Interleaver/1
  General Block Interleaver/1 -> General Block Interleaver1/1
  General Block Interleaver1/1 -> Rectangular QAM Modulator Baseband/1

== system ieee80211n/training sequence4/Modulator/Group into OFDM symbols ==
  in1 : Inport  Port=1  LatchInput=off
  in : Inport  Port=2  LatchInput=off
  Assemble Subcarriers : simulink/Math Operations/Matrix Concatenation  numInports=13  catMethod=Vertical
  DC value : Subsystem
      mask Display: disp('Zero DC')
  DC value1 : Subsystem
      mask Display: disp('Zeros, LB')
  DC value2 : Subsystem
      mask Display: disp('Zeros, UB')
  Gain : Gain  Gain=-1  SaturateOnIntegerOverflow=on
  Select data blocks : S-Function  AncestorBlock=dspindex/Multiport Selector  FunctionName=sdspmultiportsel  Parameters=rowsOrCols, numOutports, flatIdxVect, flatLenVect, idxErrMode  mask(Multiport Selector){rowsOrCols=Rows, idxCellArray={1:5, 6:18, 19:24, 25:30, 31:43, 44:48}, idxErrMode=Clip Index}
      mask prompts: rowsOrCols "Select:"; idxCellArray "Indices to output:"; idxErrMode "Invalid index:"
      mask help: Output specified rows or columns to one or more output ports. The number of output ports is determined by the number of index vectors, each specified as a separate vector entry in a cell array. Indices are 1-based and need not be unique.
      mask init:
      | [numOutports, flatLenVect, flatIdxVect] = dspblkmultiportsel(idxCellArray);
      mask Help: web(dspbhelp);
      mask StyleString: popup(Rows|Columns),edit,popup(Clip Index|Clip and Warn|Generate Error)
      mask Display: disp(['Select\n' &1]);
  Select pilots : S-Function  AncestorBlock=dspindex/Multiport Selector  FunctionName=sdspmultiportsel  Parameters=rowsOrCols, numOutports, flatIdxVect, flatLenVect, idxErrMode  mask(Multiport Selector){rowsOrCols=Columns, idxCellArray={1:params.OFDM_LSIG_SymPerFrame}, idxErrMode=Clip Index}
      mask prompts: rowsOrCols "Select:"; idxCellArray "Indices to output:"; idxErrMode "Invalid index:"
      mask help: Output specified rows or columns to one or more output ports. The number of output ports is determined by the number of index vectors, each specified as a separate vector entry in a cell array. Indices are 1-based and need not be unique.
      mask init:
      | [numOutports, flatLenVect, flatIdxVect] = dspblkmultiportsel(idxCellArray);
      mask Help: web(dspbhelp);
      mask StyleString: popup(Rows|Columns),edit,popup(Clip Index|Clip and Warn|Generate Error)
      mask Display: disp(['Select\n' &1]);
  out : Outport
  wires:
  Select data blocks/1 -> Assemble Subcarriers/2
  Select data blocks/2 -> Assemble Subcarriers/4
  Select data blocks/3 -> Assemble Subcarriers/6
  Select data blocks/4 -> Assemble Subcarriers/8
  Select data blocks/5 -> Assemble Subcarriers/10
  Select data blocks/6 -> Assemble Subcarriers/12
  Gain/1 -> Assemble Subcarriers/11
  Select pilots/1 -> Gain/1, Assemble Subcarriers/9, Assemble Subcarriers/5, Assemble Subcarriers/3
  Assemble Subcarriers/1 -> out/1
  DC value/1(out) -> Assemble Subcarriers/7
  in/1 -> Select data blocks/1
  in1/1 -> Select pilots/1
  DC value1/1(out) -> Assemble Subcarriers/1
  DC value2/1(out) -> Assemble Subcarriers/13

== system ieee80211n/training sequence4/Modulator/Modulator 1 ==
  txdata : Inport  Port=1  LatchInput=off
  Convolutional Encoder1 : commcnvcod2/Convolutional Encoder  trellis=trellisStructure  reset=None
  Gain1 : Gain  SaturateOnIntegerOverflow=on
  General Block Interleaver : commblkintrlv2/General Block Interleaver  elements=interleaverElements
  Matrix Interleaver : commblkintrlv2/Matrix Interleaver  Nrows=interleaverRows  Ncols=interleaverCols
  P2 Puncture : commsequence2/Puncture  punctureVector=punctureVector
  Rectangular QAM Modulator Baseband : commdigbbndam2/Rectangular QAM Modulator Baseband  M=modOrder  InType=Bit  Enc=Gray  PowType=Average Power  MinDist=2  AvgPow=1  PeakPow=1  Ph=0  numSamp=1
  Zero Pad : dspsigops/Zero Pad  padSigAt=End  zpadAlong=Columns  padNumOutRowsSpecMethod=User-specified  numOutRows=bitsPerBlock  padNumOutColsSpecMethod=User-specified  numOutCols=1  trunc_flag=None
      settings: AttributesFormatString=\n
  txsig : Outport
  wires:
  Rectangular QAM Modulator Baseband/1 -> Gain1/1
  Gain1/1 -> txsig/1
  txdata/1 -> Zero Pad/1
  Convolutional Encoder1/1 -> P2 Puncture/1
  Matrix Interleaver/1 -> General Block Interleaver/1
  P2 Puncture/1 -> Matrix Interleaver/1
  General Block Interleaver/1 -> Rectangular QAM Modulator Baseband/1
  Zero Pad/1 -> Convolutional Encoder1/1
